simulink model "controller"  (R2024a)
settings: Solver=VariableStepAuto  StartTime=0.0  StopTime=1  RelTol=1e-3
libraries: spsThreePhaseSeriesRLCLoadLib x3, spsThreePhaseBreakerLib x3, spsPower3phInstantaneousLib x1, spsThreePhaseParallelRLCLoadLib x1, spsThreePhaseVIMeasurementLib x1, spsThreePhaseSourceLib x1, spspowerguiLib x1
settings Model: Creator=User  LastModifiedBy=User

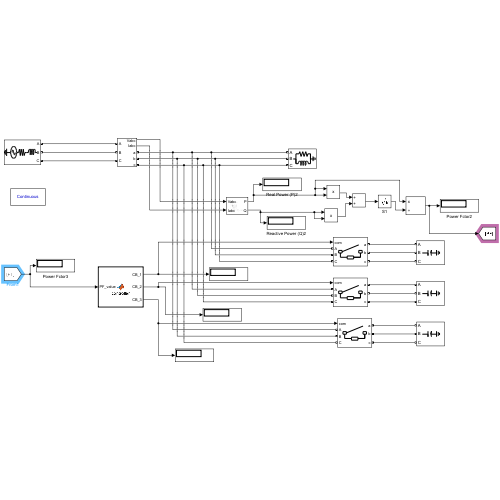
[thumbnail: Simulink's stored preview of the top-level diagram]
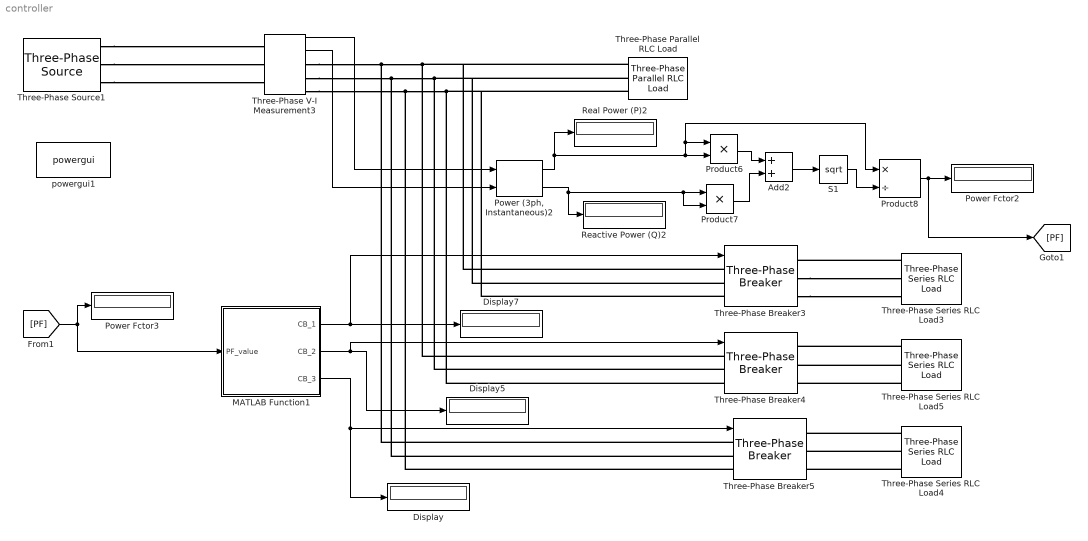
== system controller ==
  Add2 : Sum
  Display : Display
  Display5 : Display
  Display7 : Display
  MATLAB Function1 : MATLAB Function  TreatAsAtomicUnit=on
  "Power (3ph, Instantaneous)2" : spsPower3phInstantaneousLib/Power (3ph, Instantaneous)
  Power Fctor2 : Display
  Power Fctor3 : Display
  Product6 : Product
  Product7 : Product
  Product8 : Product  Inputs=*/
  Reactive Power (Q)2 : Display
  Real Power (P)2 : Display
  S1 : Sqrt
  Three-Phase Parallel RLC Load : spsThreePhaseParallelRLCLoadLib/Three-Phase Parallel RLC Load  LConnTagsString=A|B|C  Configuration=Y (grounded)  NominalVoltage=400  Vabc=[1e3 1e3 1e3]  Vabcp=[1e3 1e3 1e3]  NominalFrequency=50  UnbalancedPower=off  ActivePower=5e3  InductivePower=7000  CapacitivePower=0  Pabc=[10e3 9e3 11e3]  QLabc=[100 90 110]  QCabc=[100 90 110]  Pabcp=[10e3 9e3 11e3]  QLabcp=[100 90 110]  QCabcp=[100 90 110]  Measurements=None  LoadType=constant PQ
  Three-Phase Series RLC Load3 : spsThreePhaseSeriesRLCLoadLib/Three-Phase Series RLC Load  LConnTagsString=A|B|C  Configuration=Y (grounded)  NominalVoltage=400  Vabc=[1e3 1e3 1e3]  Vabcp=[1e3 1e3 1e3]  NominalFrequency=50  UnbalancedPower=off  ActivePower=0  InductivePower=0  CapacitivePower=1.5e3  Pabc=[10e3 9e3 11e3]  QLabc=[100 90 110]  QCabc=[100 90 110]  Pabcp=[10e3 9e3 11e3]  QLabcp=[100 90 110]  QCabcp=[100 90 110]  Measurements=None  LoadType=constant Z
  Three-Phase Series RLC Load4 : spsThreePhaseSeriesRLCLoadLib/Three-Phase Series RLC Load  LConnTagsString=A|B|C  Configuration=Y (grounded)  NominalVoltage=400  Vabc=[1e3 1e3 1e3]  Vabcp=[1e3 1e3 1e3]  NominalFrequency=50  UnbalancedPower=off  ActivePower=0  InductivePower=0  CapacitivePower=3.5e3  Pabc=[10e3 9e3 11e3]  QLabc=[100 90 110]  QCabc=[100 90 110]  Pabcp=[10e3 9e3 11e3]  QLabcp=[100 90 110]  QCabcp=[100 90 110]  Measurements=None  LoadType=constant Z
  Three-Phase Series RLC Load5 : spsThreePhaseSeriesRLCLoadLib/Three-Phase Series RLC Load  LConnTagsString=A|B|C  Configuration=Y (grounded)  NominalVoltage=400  Vabc=[1e3 1e3 1e3]  Vabcp=[1e3 1e3 1e3]  NominalFrequency=50  UnbalancedPower=off  ActivePower=0  InductivePower=0  CapacitivePower=2e3  Pabc=[10e3 9e3 11e3]  QLabc=[100 90 110]  QCabc=[100 90 110]  Pabcp=[10e3 9e3 11e3]  QLabcp=[100 90 110]  QCabcp=[100 90 110]  Measurements=None  LoadType=constant Z
  Three-Phase V-I Measurement3 : spsThreePhaseVIMeasurementLib/Three-Phase V-I Measurement  VoltageMeasurement=phase-to-ground  SetLabelV=off  LabelV=Vabc  Vpu=off  VpuLL=off  CurrentMeasurement=yes  SetLabelI=off  LabelI=Iabc  Ipu=off  Pbase=100e6  Vbase=500e3  OutputType=Complex  PhasorSimulation=off  PSBequivalent=0
  Three-Phase Breaker3 : spsThreePhaseBreakerLib/Three-Phase Breaker  InitialState=open  SwitchA=on  SwitchB=on  SwitchC=on  SwitchTimes="[1/60  5/60]"  External=on  BreakerResistance=0.01  SnubberResistance=1e6  SnubberCapacitance=inf  Measurements=None
  Three-Phase Breaker4 : spsThreePhaseBreakerLib/Three-Phase Breaker  InitialState=open  SwitchA=on  SwitchB=on  SwitchC=on  SwitchTimes="[1/60  5/60]"  External=on  BreakerResistance=0.01  SnubberResistance=1e6  SnubberCapacitance=inf  Measurements=None
  Three-Phase Breaker5 : spsThreePhaseBreakerLib/Three-Phase Breaker  InitialState=open  SwitchA=on  SwitchB=on  SwitchC=on  SwitchTimes="[1/60  5/60]"  External=on  BreakerResistance=0.01  SnubberResistance=1e6  SnubberCapacitance=inf  Measurements=None
  Three-Phase Source1 : spsThreePhaseSourceLib/Three-Phase Source  InternalConnection=Yg  VoltagePhases=off  Voltage=400  PhaseAngle=0  Voltage_phases=[25e3 25e3 25e3]/sqrt(3)  PhaseAngles_phases=[0 -120 +120]  Frequency=50  NonIdealSource=on  SpecifyImpedance=off  Resistance=0.8929  Inductance=16.58e-3  ShortCircuitLevel=1200  BaseVoltage=400  XRratio=7  BusType=swing  Pref=10e3  Qref=0  Prefabc=[10e3, 10e3, 10e3]  Qrefabc=[0, 0, 0]  Qmin=-inf  Qmax=inf
  powergui1 : spspowerguiLib/powergui  Priority=1  SimulationMode=Continuous  SampleTime=50e-6  frequency=60  Iterations=50  frequencyindice=50  Pbase=100e6  ErrMax=1e-4  UnitsV=kV  UnitsW=MW  buscounter=0  FunctionMessages=off  echomessages=off  EnableUseOfTLC=off  CurrentSourceSwitches=off  DisableSnubberDevices=off  DisableRonSwitches=off  DisableVfSwitches=off  DisplayEquations=off  AutomaticDiscreteSolvers=off  SolverType=Tustin/Backward Euler (TBE)  Interpol=off  ExternalGateDelay=off  methode=off  Ts=100  x0status=blocks  SPID=on  SwTol=0  HookPort=off  NonlinearTolerance=1e-4  nMaxIteration=100  ContinueOnMaxIteration=off  RestoreLinks=warning  ResistiveCurrentMeasurement=off  Frange=[0:2:500]  Ylog=off  Xlog=on  ShowGrid=off  save=off  variable=ZData  structure=0  ZoomFFT=off  StartTime=0.0  cycles=1  DisplayStyle=1  fundamental=60  FreqAxis=off  MaxFrequency=1000  frequencyindicesteady=1  RmsSteady=1  display=off
  wires:
  Product8/1 -> [PF], Power Fctor2/1
  Product7/1 -> Add2/2
  S1/1 -> Product8/2
  Three-Phase V-I Measurement3/2 -> "Power (3ph, Instantaneous)2"/2
  "Power (3ph, Instantaneous)2"/1 -> Real Power (P)2/1, Product8/1, Product6/1, Product6/2
  Three-Phase V-I Measurement3/1 -> "Power (3ph, Instantaneous)2"/1
  "Power (3ph, Instantaneous)2"/2 -> Reactive Power (Q)2/1, Product7/2, Product7/1
  Product6/1 -> Add2/1
  MATLAB Function1/3(CB_3) -> Display/1, Three-Phase Breaker5/1
  MATLAB Function1/2(CB_2) -> Display5/1, Three-Phase Breaker4/1
  [PF] -> MATLAB Function1/1(PF_value), Power Fctor3/1
  Add2/1 -> S1/1
  MATLAB Function1/1(CB_1) -> Display7/1, Three-Phase Breaker3/1
  connections:
  Three-Phase V-I Measurement3/RConn2 -- Three-Phase Breaker5/LConn2 -- Three-Phase Breaker4/LConn2 -- Three-Phase Parallel RLC Load/LConn2 -- Three-Phase Breaker3/LConn2
  Three-Phase V-I Measurement3/RConn3 -- Three-Phase Breaker3/LConn3 -- Three-Phase Parallel RLC Load/LConn3 -- Three-Phase Breaker4/LConn3 -- Three-Phase Breaker5/LConn3
  Three-Phase V-I Measurement3/RConn1 -- Three-Phase Breaker3/LConn1 -- Three-Phase Parallel RLC Load/LConn1 -- Three-Phase Breaker4/LConn1 -- Three-Phase Breaker5/LConn1
  Three-Phase Series RLC Load5/LConn1 -- Three-Phase Breaker4/RConn1
  Three-Phase Source1/RConn1 -- Three-Phase V-I Measurement3/LConn1
  Three-Phase Source1/RConn3 -- Three-Phase V-I Measurement3/LConn3
  Three-Phase Series RLC Load5/LConn2 -- Three-Phase Breaker4/RConn2
  Three-Phase Breaker3/RConn2 -- Three-Phase Series RLC Load3/LConn2
  Three-Phase Source1/RConn2 -- Three-Phase V-I Measurement3/LConn2
  Three-Phase Series RLC Load5/LConn3 -- Three-Phase Breaker4/RConn3
  Three-Phase Series RLC Load4/LConn3 -- Three-Phase Breaker5/RConn3
  Three-Phase Series RLC Load4/LConn1 -- Three-Phase Breaker5/RConn1
  Three-Phase Series RLC Load4/LConn2 -- Three-Phase Breaker5/RConn2
  Three-Phase Series RLC Load3/LConn1 -- Three-Phase Breaker3/RConn1
  Three-Phase Breaker3/RConn3 -- Three-Phase Series RLC Load3/LConn3

== matlab function controller/MATLAB Function1 ==
  data: PF_value input; CB_1 output; CB_2 output; CB_3 output
function [CB_1,CB_2,CB_3] = controller(PF_value)

if (PF_value<=0.60)
    CB_1=1;
    CB_2=0;
    CB_3=0;

elseif (PF_value<=0.75)
    CB_1=0;
    CB_2=1;
    CB_3=0;

elseif (PF_value<=0.85)
    CB_1=0;
    CB_2=0;
    CB_3=1;
else 
    CB_1=0;
    CB_2=0;
    CB_3=1;
end

end
